simulink library "fixpt_megmaFuncBlkhidden1"  (Simulink 5.0)
libraries: funcsetup x5, fixpt_lib_3p1 x5, fixpt_megmaFuncBlkhidden1 x2
settings Model: Creator=krishnan  LastModifiedBy=krishnan  ExtModeAutoUpdateStatusClock=off

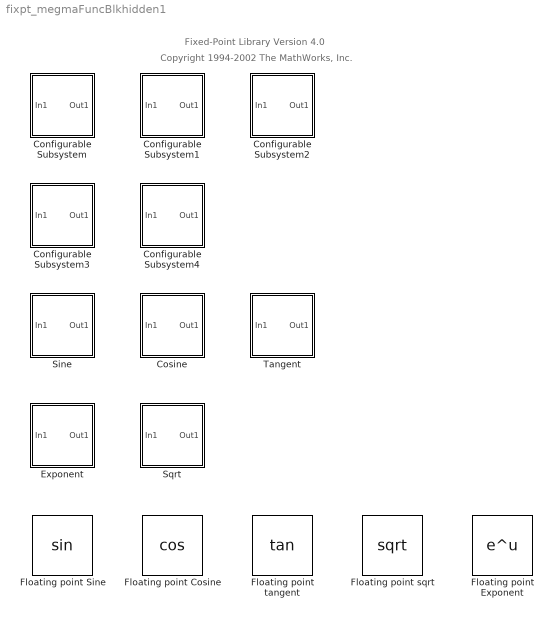
== system fixpt_megmaFuncBlkhidden1 ==
  note: Fixed-Point Library Version 4.0
  note: Copyright 1994-2002 The MathWorks, Inc.
  Configurable Subsystem : Subsystem  BlockChoice=Floating point Sine
      settings: TemplateBlock=self  MemberBlocks=Floating point Sine,Sine
  Configurable Subsystem1 : Subsystem  BlockChoice=Cosine
      settings: TemplateBlock=self  MemberBlocks=Cosine,Floating point Cosine
  Configurable Subsystem2 : Subsystem  BlockChoice=Floating point tangent
      settings: TemplateBlock=self  MemberBlocks=Floating point tangent,Tangent
  Configurable Subsystem3 : Subsystem  BlockChoice=Exponent
      settings: TemplateBlock=self  MemberBlocks=Exponent,Floating point Exponent
  Configurable Subsystem4 : Subsystem  BlockChoice=Floating point sqrt
      settings: TemplateBlock=self  MemberBlocks=Floating point sqrt,Sqrt
  Cosine : Subsystem  mask(MEGMA Fixed-Point Cosine){yData=[1 2 3], xData=[1 2 3], Recompute=Compute always, yData_nonvisible=, xData_nonvisible=, Spacing_nonvisible=, Nptsmax_nonvisible=, ErrMax_nonvisible=, RndMeth_nonvisible=, yScale_nonvisible=, yDt_nonvisible=, xScale_nonvisible=, xDt_nonvisible=, xMax_nonvisible=, xMin_nonvisible=, Spacing='pow2', Nptsmax=[], ErrMax=0.01, RndMeth='floor', yScale=2^-5, xScale=2^-5, yDt=sfix(16), xDt=sfix(16), xmax=2*pi, xmin=0}
      mask prompts: Recompute "Lookup table breakpoints"; Spacing "Allowed spacing 'pow2','even', or 'unrestricted'(default)"; Nptsmax "Maximum number of breakpoints"; ErrMax "Maximum worst case approximation error"; RndMeth "Rounding method 'floor'(default),'ceil','near' or 'zero'"; yScale "Output Scaling"; xScale "Input Scaling"; yDt "Output Datatype"; xDt "Input Datatype"; xmax "Maximum input value of interest"; xmin "Minimum input value of interest"
      mask help: MEGMA Cosine
      mask init:
      | FuncStr = 'cos(x)';
      | if Recompute ~= 3
      |  [xData,yData]= fixpt_look1_func_approx(FuncStr,xmin,xmax,xDt,xScale,yDt,yScale,RndMeth,ErrMax,Nptsmax,Spacing,Recompute);
      | end
      mask Help: web(fpbhelp('cosine'));
      mask StyleString: edit,edit,popup(Compute Always|Cache for a specific MATLAB session|Cache across different MATLAB sessions),edit,edit,edit,edit,edit,edit,edit,edit,edit,edit,edit,edit,edit,edit,edit,edit,edit,edit,edit,edit,edit,edit
      mask Display: disp('y=cos(x)')
  Exponent : Subsystem  mask(MEGMA Fixed-Point Exponent){yData=[1 2 3], xData=[1 2 3], Recompute=Compute always, yData_nonvisible=, xData_nonvisible=, Spacing_nonvisible=, Nptsmax_nonvisible=, ErrMax_nonvisible=, RndMeth_nonvisible=, yScale_nonvisible=, yDt_nonvisible=, xScale_nonvisible=, xDt_nonvisible=, xMax_nonvisible=, xMin_nonvisible=, Spacing='pow2', Nptsmax=[], ErrMax=0.01, RndMeth='floor', yScale=2^-5, xScale=2^-5, yDt=sfix(16), xDt=sfix(16), xmax=2*pi, xmin=0}
      mask prompts: Recompute "Lookup table breakpoints"; Spacing "Allowed spacing 'pow2','even', or 'unrestricted'(default)"; Nptsmax "Maximum number of breakpoints"; ErrMax "Maximum worst case approximation error"; RndMeth "Rounding method 'floor'(default),'ceil','near' or 'zero'"; yScale "Output Scaling"; xScale "Input Scaling"; yDt "Output Datatype"; xDt "Input Datatype"; xmax "Maximum input value of interest"; xmin "Minimum input value of interest"
      mask help: MEGMA Exponent
      mask init:
      | FuncStr = 'exp(x)';
      | if Recompute ~= 3
      |  [xData,yData]= fixpt_look1_func_approx(FuncStr,xmin,xmax,xDt,xScale,yDt,yScale,RndMeth,ErrMax,Nptsmax,Spacing,Recompute);
      | end
      mask Help: web(fpbhelp('exponent'));
      mask StyleString: edit,edit,popup(Compute Always|Cache for a specific MATLAB session|Cache across different MATLAB sessions),edit,edit,edit,edit,edit,edit,edit,edit,edit,edit,edit,edit,edit,edit,edit,edit,edit,edit,edit,edit,edit,edit
      mask Display: disp('y=exp(x)')
  Floating point Cosine : Trigonometry  Operator=cos
  Floating point Exponent : Math
  Floating point Sine : Trigonometry
  Floating point sqrt : Math  Operator=sqrt
  Floating point tangent : Trigonometry  Operator=tan
  Sine : Subsystem  mask(MEGMA Fixed-Point Sine){yData=[1 2 3], xData=[1 2 3], Recompute=Compute always, yData_nonvisible=, xData_nonvisible=, Spacing_nonvisible=, Nptsmax_nonvisible=, ErrMax_nonvisible=, RndMeth_nonvisible=, yScale_nonvisible=, yDt_nonvisible=, xScale_nonvisible=, xDt_nonvisible=, xMax_nonvisible=, xMin_nonvisible=, Spacing='pow2', Nptsmax=[], ErrMax=0.01, RndMeth='floor', yScale=2^-5, xScale=2^-5, yDt=sfix(16), xDt=sfix(16), xmax=2*pi, xmin=0}
      mask prompts: Recompute "Lookup table breakpoints"; Spacing "Allowed spacing 'pow2','even', or 'unrestricted'(default)"; Nptsmax "Maximum number of breakpoints"; ErrMax "Maximum worst case approximation error"; RndMeth "Rounding method 'floor'(default),'ceil','near' or 'zero'"; yScale "Output Scaling"; xScale "Input Scaling"; yDt "Output Datatype"; xDt "Input Datatype"; xmax "Maximum input value of interest"; xmin "Minimum input value of interest"
      mask help: MEGMA Sine
      mask init:
      | FuncStr = 'sin(x)';
      | if Recompute ~= 3
      |  [xData,yData]= fixpt_look1_func_approx(FuncStr,xmin,xmax,xDt,xScale,yDt,yScale,RndMeth,ErrMax,Nptsmax,Spacing,Recompute);
      | end
      mask Help: web(fpbhelp('sine'));
      mask StyleString: edit,edit,popup(Compute Always|Cache for a specific MATLAB session|Cache across different MATLAB sessions),edit,edit,edit,edit,edit,edit,edit,edit,edit,edit,edit,edit,edit,edit,edit,edit,edit,edit,edit,edit,edit,edit
      mask Display: disp('y=sin(x)')
  Sqrt : Subsystem  mask(MEGMA Fixed-Point Sqrt){yData=[1 2 3], xData=[1 2 3], Recompute=Compute always, yData_nonvisible=, xData_nonvisible=, Spacing_nonvisible=, Nptsmax_nonvisible=, ErrMax_nonvisible=, RndMeth_nonvisible=, yScale_nonvisible=, yDt_nonvisible=, xScale_nonvisible=, xDt_nonvisible=, xMax_nonvisible=, xMin_nonvisible=, Spacing='pow2', Nptsmax=[], ErrMax=0.01, RndMeth='floor', yScale=2^-5, xScale=2^-5, yDt=sfix(16), xDt=sfix(16), xmax=2*pi, xmin=0}
      mask prompts: Recompute "Lookup table breakpoints"; Spacing "Allowed spacing 'pow2','even', or 'unrestricted'(default)"; Nptsmax "Maximum number of breakpoints"; ErrMax "Maximum worst case approximation error"; RndMeth "Rounding method 'floor'(default),'ceil','near' or 'zero'"; yScale "Output Scaling"; xScale "Input Scaling"; yDt "Output Datatype"; xDt "Input Datatype"; xmax "Maximum input value of interest"; xmin "Minimum input value of interest"
      mask help: MEGMA Sqrt
      mask init:
      | FuncStr = 'sqrt(x)';
      | if Recompute ~= 3
      |  [xData,yData]= fixpt_look1_func_approx(FuncStr,xmin,xmax,xDt,xScale,yDt,yScale,RndMeth,ErrMax,Nptsmax,Spacing,Recompute);
      | end
      mask Help: web(fpbhelp('sqrt'));
      mask StyleString: edit,edit,popup(Compute Always|Cache for a specific MATLAB session|Cache across different MATLAB sessions),edit,edit,edit,edit,edit,edit,edit,edit,edit,edit,edit,edit,edit,edit,edit,edit,edit,edit,edit,edit,edit,edit
      mask Display: disp('y=sqrt(x)')
  Tangent : Subsystem  mask(MEGMA Fixed-Point Tangent){yData=[1 2 3], xData=[1 2 3], Recompute=Compute always, yData_nonvisible=, xData_nonvisible=, Spacing_nonvisible=, Nptsmax_nonvisible=, ErrMax_nonvisible=, RndMeth_nonvisible=, yScale_nonvisible=, yDt_nonvisible=, xScale_nonvisible=, xDt_nonvisible=, xMax_nonvisible=, xMin_nonvisible=, Spacing='pow2', Nptsmax=[], ErrMax=0.01, RndMeth='floor', yScale=2^-5, xScale=2^-5, yDt=sfix(16), xDt=sfix(16), xmax=2*pi, xmin=0}
      mask prompts: Recompute "Lookup table breakpoints"; Spacing "Allowed spacing 'pow2','even', or 'unrestricted'(default)"; Nptsmax "Maximum number of breakpoints"; ErrMax "Maximum worst case approximation error"; RndMeth "Rounding method 'floor'(default),'ceil','near' or 'zero'"; yScale "Output Scaling"; xScale "Input Scaling"; yDt "Output Datatype"; xDt "Input Datatype"; xmax "Maximum input value of interest"; xmin "Minimum input value of interest"
      mask help: MEGMA Tangent
      mask init:
      | FuncStr = 'tan(x)';
      | if Recompute ~= 3
      |  [xData,yData]= fixpt_look1_func_approx(FuncStr,xmin,xmax,xDt,xScale,yDt,yScale,RndMeth,ErrMax,Nptsmax,Spacing,Recompute);
      | end
      mask Help: web(fpbhelp('tangent'));
      mask StyleString: edit,edit,popup(Compute Always|Cache for a specific MATLAB session|Cache across different MATLAB sessions),edit,edit,edit,edit,edit,edit,edit,edit,edit,edit,edit,edit,edit,edit,edit,edit,edit,edit,edit,edit,edit,edit
      mask Display: disp('y=tan(x)')

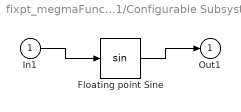
== system fixpt_megmaFuncBlkhidden1/Configurable Subsystem ==
  In1 : Inport
  Floating point Sine : Trigonometry
  Out1 : Outport
  wires:
  In1/1 -> Floating point Sine/1
  Floating point Sine/1 -> Out1/1

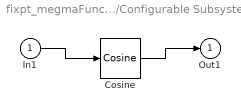
== system fixpt_megmaFuncBlkhidden1/Configurable Subsystem1 ==
  In1 : Inport
  Cosine : fixpt_megmaFuncBlkhidden1/Cosine  yData=[1 2 3]  xData=[1 2 3]  Recompute=Compute Always  yData_nonvisible=[1;0.999511758485136;0.998047510700099;0.995608686458002;0.992197667229329;0.987817783816472;0.982473313101255;0.976169473868635;0.968912421710645;0.960709243015562;0.951567948048172;0.941497463127881;0.930507621912314;0.918609155794918;0.905813683425936;0.892133699366994;0.877582561890373;0.86217447993488;0.845924499231068;0.828848487609326;0.810963119505218;0.792285859677179;0.772834946152472;0.752629372418066;0.731688868873821;0.71003388356608;0.687685562220505;0.664665727593633;0.640996858163325;0.616702066178912;0.591805075092477;0.566330196393309;0.54030230586814;0.513746819310368;0.486689667701963;0.459157271892304;0.431176516798666;0.402774725153557;0.373979630824533;0.344819351732545;0.315322362395269;0.28551746612222;0.255433766888812;0.225100640916817;0.194547707988987;0.163804802525833;0.132901944452825;0.101869309886441;0.0707372016677029;0.0395360197719658;0.00829623162385838;-0.0229516576536404;-0.0541771350269363;-0.0853497093472792;-0.116438941124852;-0.147414472252418;-0.178246055649492;-0.208903584798109;-0.239357123141322;-0.269576933315742;-0.299533506189574;-0.329197589677777;-0.358540217306233;-0.387532736497014;-0.416146836547142;-0.444354576273508;-0.47212841129696;-0.499441220938929;-0.526266334704305;-0.552577558324725;-0.578349199336833;-0.603556092170533;-0.628173622722739;-0.652177752392634;-0.675545041554953;-0.698252672448376;-0.720278471456692;-0.741600930760952;-0.762199229341495;-0.782053253309314;-0.801143615546934;-0.819451674639598;-0.836959553078294;-0.853650154716842;-0.869507181465984;-0.884515149208199;-0.898659402917676;-0.911926130970699;-0.924302378632464;-0.935776060707157;-0.946335973338945;-0.955971804952348;-0.964674146321316;-0.972434499757186;-0.979245287406521;-0.985099858650763;-0.989992496600445;-0.993918423677641;-0.996873806281181;-0.998855758530109;-0.999862345081687;-0.999892583021229;-0.9989464428219;-0.99702484837355;-0.994129676080546;-0.990263753029502;-0.98543085422867;-0.979635698921714;-0.972883945979446;-0.965182188374036;-0.956537946741083;-0.946959662035847;-0.936456687290796;-0.925039278482532;-0.912718584516998;-0.899506636342767;-0.88541633520302;-0.870461440037704;-0.85465655404816;-0.838017110437342;-0.820559357339561;-0.802300341954454;-0.783257893900684;-0.76345060780562;-0.742897825147999;-0.721619615371299;-0.699636756286272;-0.676970713781757;-0.653643620863612;-0.629678256042204;-0.605098021089583;-0.579926918188046;-0.554189526492417;-0.527910978128915;-0.501116933654064;-0.47383355699759;-0.446087489913793;-0.417905825966321;-0.38931608407177;-0.360346181627922;-0.331024407252887;-0.301379393161745;-0.271440087207671;-0.24123572461485;-0.21079579943078;-0.180150035725827;-0.149328358568183;-0.118360864802541;-0.0872777936610349;-0.0561094972351469;-0.0248864108374021;0.00636097671819611;0.0376021528879766;0.0688066111935807;0.0999438810110212;0.130983557324729;0.161895330417537;0.192649015467599;0.223214582023364;0.253562183327795;0.283662185463226;0.313485196288377;0.343002094139282;0.372184056266098;0.401002586978036;0.429429545468913;0.457437173296176;0.484998121486549;0.512085477241841;0.538672790218836;0.564734098357607;0.590243953233023;0.615177444904708;0.639510226241173;0.663218536694376;0.686279225501496;0.70866977429126;0.730368319072748;0.751353671585211;0.771605339988047;0.791103548870739;0.809829258563201;0.827764183727699;0.844890811214172;0.861192417161521;0.876653083328182;0.891257712636015;0.904992043912346;0.917842665815758;0.929797029932041;0.940843463027505;0.950971178447692;0.960170286650366;0.968431804862477;0.975747665851692;0.982110725803907;0.987514771299061;0.991954525378437;0.995425652697519;0.997924763759387;0.999449418224499;0.999998127293645]  xData_nonvisible=[0;0.03125;0.0625;0.09375;0.125;0.15625;0.1875;0.21875;0.25;0.28125;0.3125;0.34375;0.375;0.40625;0.4375;0.46875;0.5;0.53125;0.5625;0.59375;0.625;0.65625;0.6875;0.71875;0.75;0.78125;0.8125;0.84375;0.875;0.90625;0.9375;0.96875;1;1.03125;1.0625;1.09375;1.125;1.15625;1.1875;1.21875;1.25;1.28125;1.3125;1.34375;1.375;1.40625;1.4375;1.46875;1.5;1.53125;1.5625;1.59375;1.625;1.65625;1.6875;1.71875;1.75;1.78125;1.8125;1.84375;1.875;1.90625;1.9375;1.96875;2;2.03125;2.0625;2.09375;2.125;2.15625;2.1875;2.21875;2.25;2.28125;2.3125;2.34375;2.375;2.40625;2.4375;2.46875;2.5;2.53125;2.5625;2.59375;2.625;2.65625;2.6875;2.71875;2.75;2.78125;2.8125;2.84375;2.875;2.90625;2.9375;2.96875;3;3.03125;3.0625;3.09375;3.125;3.15625;3.1875;3.21875;3.25;3.28125;3.3125;3.34375;3.375;3.40625;3.4375;3.46875;3.5;3.53125;3.5625;3.59375;3.625;3.65625;3.6875;3.71875;3.75;3.78125;3.8125;3.84375;3.875;3.90625;3.9375;3.96875;4;4.03125;4.0625;4.09375;4.125;4.15625;4.1875;4.21875;4.25;4.28125;4.3125;4.34375;4.375;4.40625;4.4375;4.46875;4.5;4.53125;4.5625;4.59375;4.625;4.65625;4.6875;4.71875;4.75;4.78125;4.8125;4.84375;4.875;4.90625;4.9375;4.96875;5;5.03125;5.0625;5.09375;5.125;5.15625;5.1875;5.21875;5.25;5.28125;5.3125;5.34375;5.375;5.40625;5.4375;5.46875;5.5;5.53125;5.5625;5.59375;5.625;5.65625;5.6875;5.71875;5.75;5.78125;5.8125;5.84375;5.875;5.90625;5.9375;5.96875;6;6.03125;6.0625;6.09375;6.125;6.15625;6.1875;6.21875;6.25;6.28125]  Spacing_nonvisible='pow2'  Nptsmax_nonvisible=[]  ErrMax_nonvisible=0.01  RndMeth_nonvisible='floor'  yScale_nonvisible=2^-5  yDt_nonvisible=sfix(16)  xScale_nonvisible=2^-5  xDt_nonvisible=sfix(16)  xMax_nonvisible=2*pi  xMin_nonvisible=0  Spacing='pow2'  Nptsmax=[]  ErrMax=0.01  RndMeth='floor'  yScale=2^-5  xScale=2^-5  yDt=sfix(16)  xDt=sfix(16)  xmax=2*pi  xmin=0
  Out1 : Outport
  wires:
  In1/1 -> Cosine/1
  Cosine/1 -> Out1/1

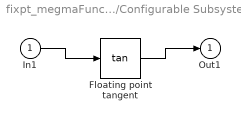
== system fixpt_megmaFuncBlkhidden1/Configurable Subsystem2 ==
  In1 : Inport
  Floating point tangent : Trigonometry  Operator=tan
  Out1 : Outport
  wires:
  In1/1 -> Floating point tangent/1
  Floating point tangent/1 -> Out1/1

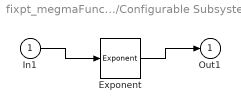
== system fixpt_megmaFuncBlkhidden1/Configurable Subsystem3 ==
  In1 : Inport
  Exponent : fixpt_megmaFuncBlkhidden1/Exponent  yData=[1 2 3]  xData=[1 2 3]  Recompute=Compute Always  yData_nonvisible=[1;1.0317434074991;1.06449445891786;1.09828514030783;1.13314845306683;1.1691184461695;1.20623024942098;1.2445201077661;1.28402541668774;1.32478475872887;1.3668379411738;1.41022603492571;1.4549914146182;1.50117780000012;1.54883029863413;1.59799544995063;1.64872127070013;1.7010573018484;1.7550546569603;1.81076607211939;1.86824595743222;1.92755045016754;1.98873746958229;2.05186677348798;2.11700001661267;2.18420081081562;2.25353478721321;2.32506966027712;2.3988752939671;2.47502376996303;2.55358945806293;2.63464908881563;2.71828182845905;2.80456935623723;2.89359594417176;2.98544853936536;3.08021684891803;3.17799342753884;3.27887376793867;3.38295639409247;3.49034295746184;3.60113833627218;3.7154507379411;3.83339180475841;3.95507672292058;4.08062433502646;4.21015725614396;4.34380199356104;4.48168907033806;4.62395315278208;4.7707331819676;4.92217250943229;5.07841903718008;5.23962536212849;5.40594892514117;5.57755216479126;5.75460267600573;5.93727337374561;6.12574266188199;6.32019460743274;6.52081912033011;6.72781213889469;6.94137582119704;7.16171874249371;7.38905609893065;7.62360991771274;7.86560927394489;8.11529051435645;8.37289748812726;8.6386817850411;8.91290298119874;9.1958288925309;9.48773583635853;9.78890890125589;10.0996422254801;10.4202392842386;10.7510131860764;11.0922869786702;11.4443939643311;11.8076780255212;12.1824939607035;12.5692078308534;12.9681973169691;13.3798520889305;13.8045741860671;14.242778409807;14.6948927287889;15.1613586968345;15.6426318841882;16.1391823224464;16.6514949636101;17.1800701537093;17.7254241214616;18.2880894824436;18.8686157592649;19.4675699182552;20.0855369231877;20.7231203065787;21.3809427591233;22.0596467378412;22.7598950935267;23.4823717181174;24.227782212611;24.9968545761854;25.7903399171931;26.6090131867249;27.4536739354601;28.3251470945409;29.2242837812349;30.1519621301721;31.1090881509677;32.0965966130693;33.1154519586923;34.166649244734;35.2512151145885;36.3702088008095;37.524723159601;38.7158857381472;39.9448598758219;41.2128458403547;42.5210820000628;43.8708460332935;45.2634561762588;46.7002725104795;48.1826982910988;49.7121813173595;51.2902153465857;52.9183415530491;54.5981500331442;56.3312813583435;58.119428177448;59.9643368696996;61.8678092503679;63.8317043304791;65.8579401324037;67.9484955630781;70.1054123466879;72.3307970187014;74.6268229832009;76.9957326355201;79.4398395522613;81.9615307508321;84.563269020706;87.2475953286865;90.0171313005218;92.8745817812945;95.8227374770869;98.8644776805016;102.0027730827;105.240688674702;108.58138674079;112.02812994692;115.584284527188;119.253323571426;123.038830417177;126.944502149322;130.974153210819;135.13171912804;139.421260354375;143.846966235843;148.413159102577;153.124298490199;157.984985495187;162.999967268501;168.174141651845;173.512561961112;179.020441921657;184.703160760245;190.56626845863;196.615491173896;202.856736830865;209.296100892025;215.939872310614;222.794539672674;229.866797534079;237.163552958717;244.69193226422;252.459287981826;260.473206037167;268.741513159002;277.272284523134;286.073851638959;295.154810486372;304.524029910962;314.190660285694;324.164142447555;334.454216917865;345.070933415282;356.024660670779;367.326096554181;378.986278522156;391.016594397853;403.428793492735;416.234998081446;429.447715240934;443.079849065385;457.144713268909;471.656044188264;486.628014198347;502.075245553524;518.012824668342;534.45631685155]  xData_nonvisible=[0;0.03125;0.0625;0.09375;0.125;0.15625;0.1875;0.21875;0.25;0.28125;0.3125;0.34375;0.375;0.40625;0.4375;0.46875;0.5;0.53125;0.5625;0.59375;0.625;0.65625;0.6875;0.71875;0.75;0.78125;0.8125;0.84375;0.875;0.90625;0.9375;0.96875;1;1.03125;1.0625;1.09375;1.125;1.15625;1.1875;1.21875;1.25;1.28125;1.3125;1.34375;1.375;1.40625;1.4375;1.46875;1.5;1.53125;1.5625;1.59375;1.625;1.65625;1.6875;1.71875;1.75;1.78125;1.8125;1.84375;1.875;1.90625;1.9375;1.96875;2;2.03125;2.0625;2.09375;2.125;2.15625;2.1875;2.21875;2.25;2.28125;2.3125;2.34375;2.375;2.40625;2.4375;2.46875;2.5;2.53125;2.5625;2.59375;2.625;2.65625;2.6875;2.71875;2.75;2.78125;2.8125;2.84375;2.875;2.90625;2.9375;2.96875;3;3.03125;3.0625;3.09375;3.125;3.15625;3.1875;3.21875;3.25;3.28125;3.3125;3.34375;3.375;3.40625;3.4375;3.46875;3.5;3.53125;3.5625;3.59375;3.625;3.65625;3.6875;3.71875;3.75;3.78125;3.8125;3.84375;3.875;3.90625;3.9375;3.96875;4;4.03125;4.0625;4.09375;4.125;4.15625;4.1875;4.21875;4.25;4.28125;4.3125;4.34375;4.375;4.40625;4.4375;4.46875;4.5;4.53125;4.5625;4.59375;4.625;4.65625;4.6875;4.71875;4.75;4.78125;4.8125;4.84375;4.875;4.90625;4.9375;4.96875;5;5.03125;5.0625;5.09375;5.125;5.15625;5.1875;5.21875;5.25;5.28125;5.3125;5.34375;5.375;5.40625;5.4375;5.46875;5.5;5.53125;5.5625;5.59375;5.625;5.65625;5.6875;5.71875;5.75;5.78125;5.8125;5.84375;5.875;5.90625;5.9375;5.96875;6;6.03125;6.0625;6.09375;6.125;6.15625;6.1875;6.21875;6.25;6.28125]  Spacing_nonvisible='pow2'  Nptsmax_nonvisible=[]  ErrMax_nonvisible=0.01  RndMeth_nonvisible='floor'  yScale_nonvisible=2^-5  yDt_nonvisible=sfix(16)  xScale_nonvisible=2^-5  xDt_nonvisible=sfix(16)  xMax_nonvisible=2*pi  xMin_nonvisible=0  Spacing='pow2'  Nptsmax=[]  ErrMax=0.01  RndMeth='floor'  yScale=2^-5  xScale=2^-5  yDt=sfix(16)  xDt=sfix(16)  xmax=2*pi  xmin=0
  Out1 : Outport
  wires:
  In1/1 -> Exponent/1
  Exponent/1 -> Out1/1

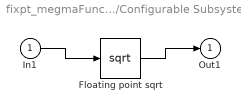
== system fixpt_megmaFuncBlkhidden1/Configurable Subsystem4 ==
  In1 : Inport
  Floating point sqrt : Math  Operator=sqrt
  Out1 : Outport
  wires:
  In1/1 -> Floating point sqrt/1
  Floating point sqrt/1 -> Out1/1

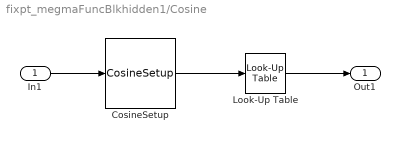
== system fixpt_megmaFuncBlkhidden1/Cosine ==
  In1 : Inport
  CosineSetup : funcsetup/CosineSetup  yData=yData  xData=xData  yData_nonvisible=yData_nonvisible  xData_nonvisible=xData_nonvisible  Spacing_nonvisible=Spacing_nonvisible  Nptsmax_nonvisible=Nptsmax_nonvisible  ErrMax_nonvisible=ErrMax_nonvisible  RndMeth_nonvisible=RndMeth_nonvisible  yScale_nonvisible=yScale_nonvisible  yDt_nonvisible=yDt_nonvisible  xScale_nonvisible=xScale_nonvisible  xDt_nonvisible=xDt_nonvisible  xMax_nonvisible=xMax_nonvisible  xMin_nonvisible=xMin_nonvisible  Spacing=Spacing  Nptsmax=Nptsmax  ErrMax=ErrMax  RndMeth=RndMeth  yScale=yScale  xScale=xScale  yDt=yDt  xDt=xDt  xmax=xmax  xmin=xmin
  Look-Up Table : fixpt_lib_3p1/LookUp/Look-Up Table  XLookUpData=xData  YLookUpData=yData  LookUpMeth=Interpolation-Use End Values  OutputDataTypeScalingMode=Specify via dialog  OutDataType=yDt  OutScaling=yScale  DoSatur=off  DblOver=off  dolog=on
  Out1 : Outport
  wires:
  CosineSetup/1 -> Look-Up Table/1
  In1/1 -> CosineSetup/1
  Look-Up Table/1 -> Out1/1

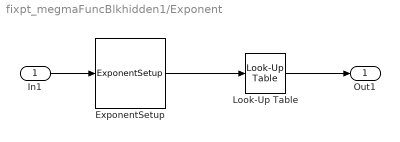
== system fixpt_megmaFuncBlkhidden1/Exponent ==
  In1 : Inport
  ExponentSetup : funcsetup/ExponentSetup  yData=yData  xData=xData  yData_nonvisible=yData_nonvisible  xData_nonvisible=xData_nonvisible  Spacing_nonvisible=Spacing_nonvisible  Nptsmax_nonvisible=Nptsmax_nonvisible  ErrMax_nonvisible=ErrMax_nonvisible  RndMeth_nonvisible=RndMeth_nonvisible  yScale_nonvisible=yScale_nonvisible  yDt_nonvisible=yDt_nonvisible  xScale_nonvisible=xScale_nonvisible  xDt_nonvisible=xDt_nonvisible  xMax_nonvisible=xMax_nonvisible  xMin_nonvisible=xMin_nonvisible  Spacing=Spacing  Nptsmax=Nptsmax  ErrMax=ErrMax  RndMeth=RndMeth  yScale=yScale  xScale=xScale  yDt=yDt  xDt=xDt  xmax=xmax  xmin=xmin
  Look-Up Table : fixpt_lib_3p1/LookUp/Look-Up Table  XLookUpData=xData  YLookUpData=yData  LookUpMeth=Interpolation-Use End Values  OutputDataTypeScalingMode=Specify via dialog  OutDataType=yDt  OutScaling=yScale  DoSatur=off  DblOver=off  dolog=on
  Out1 : Outport
  wires:
  ExponentSetup/1 -> Look-Up Table/1
  In1/1 -> ExponentSetup/1
  Look-Up Table/1 -> Out1/1

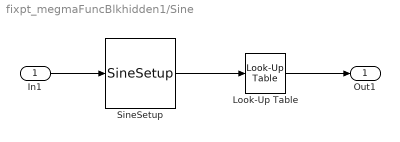
== system fixpt_megmaFuncBlkhidden1/Sine ==
  In1 : Inport
  Look-Up Table : fixpt_lib_3p1/LookUp/Look-Up Table  XLookUpData=xData  YLookUpData=yData  LookUpMeth=Interpolation-Use End Values  OutputDataTypeScalingMode=Specify via dialog  OutDataType=yDt  OutScaling=yScale  DoSatur=off  DblOver=off  dolog=on
  SineSetup : funcsetup/SineSetup  yData=yData  xData=xData  yData_nonvisible=yData_nonvisible  xData_nonvisible=xData_nonvisible  Spacing_nonvisible=Spacing_nonvisible  Nptsmax_nonvisible=Nptsmax_nonvisible  ErrMax_nonvisible=ErrMax_nonvisible  RndMeth_nonvisible=RndMeth_nonvisible  yScale_nonvisible=yScale_nonvisible  yDt_nonvisible=yDt_nonvisible  xScale_nonvisible=xScale_nonvisible  xDt_nonvisible=xDt_nonvisible  xMax_nonvisible=xMax_nonvisible  xMin_nonvisible=xMin_nonvisible  Spacing=Spacing  Nptsmax=Nptsmax  ErrMax=ErrMax  RndMeth=RndMeth  yScale=yScale  xScale=xScale  yDt=yDt  xDt=xDt  xmax=xmax  xmin=xmin
  Out1 : Outport
  wires:
  Look-Up Table/1 -> Out1/1
  In1/1 -> SineSetup/1
  SineSetup/1 -> Look-Up Table/1

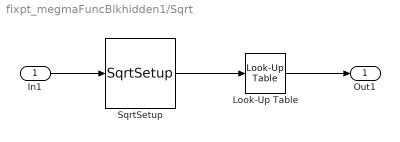
== system fixpt_megmaFuncBlkhidden1/Sqrt ==
  In1 : Inport
  Look-Up Table : fixpt_lib_3p1/LookUp/Look-Up Table  XLookUpData=xData  YLookUpData=yData  LookUpMeth=Interpolation-Use End Values  OutputDataTypeScalingMode=Specify via dialog  OutDataType=yDt  OutScaling=yScale  DoSatur=off  DblOver=off  dolog=on
  SqrtSetup : funcsetup/SqrtSetup  yData=yData  xData=xData  yData_nonvisible=yData_nonvisible  xData_nonvisible=xData_nonvisible  Spacing_nonvisible=Spacing_nonvisible  Nptsmax_nonvisible=Nptsmax_nonvisible  ErrMax_nonvisible=ErrMax_nonvisible  RndMeth_nonvisible=RndMeth_nonvisible  yScale_nonvisible=yScale_nonvisible  yDt_nonvisible=yDt_nonvisible  xScale_nonvisible=xScale_nonvisible  xDt_nonvisible=xDt_nonvisible  xMax_nonvisible=xMax_nonvisible  xMin_nonvisible=xMin_nonvisible  Spacing=Spacing  Nptsmax=Nptsmax  ErrMax=ErrMax  RndMeth=RndMeth  yScale=yScale  xScale=xScale  yDt=yDt  xDt=xDt  xmax=xmax  xmin=xmin
  Out1 : Outport
  wires:
  Look-Up Table/1 -> Out1/1
  In1/1 -> SqrtSetup/1
  SqrtSetup/1 -> Look-Up Table/1

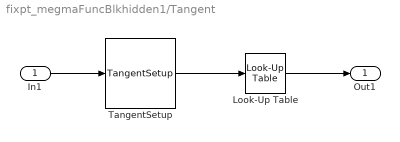
== system fixpt_megmaFuncBlkhidden1/Tangent ==
  In1 : Inport
  Look-Up Table : fixpt_lib_3p1/LookUp/Look-Up Table  XLookUpData=xData  YLookUpData=yData  LookUpMeth=Interpolation-Use End Values  OutputDataTypeScalingMode=Specify via dialog  OutDataType=yDt  OutScaling=yScale  DoSatur=off  DblOver=off  dolog=on
  TangentSetup : funcsetup/TangentSetup  yData=yData  xData=xData  yData_nonvisible=yData_nonvisible  xData_nonvisible=xData_nonvisible  Spacing_nonvisible=Spacing_nonvisible  Nptsmax_nonvisible=Nptsmax_nonvisible  ErrMax_nonvisible=ErrMax_nonvisible  RndMeth_nonvisible=RndMeth_nonvisible  yScale_nonvisible=yScale_nonvisible  yDt_nonvisible=yDt_nonvisible  xScale_nonvisible=xScale_nonvisible  xDt_nonvisible=xDt_nonvisible  xMax_nonvisible=xMax_nonvisible  xMin_nonvisible=xMin_nonvisible  Spacing=Spacing  Nptsmax=Nptsmax  ErrMax=ErrMax  RndMeth=RndMeth  yScale=yScale  xScale=xScale  yDt=yDt  xDt=xDt  xmax=xmax  xmin=xmin
  Out1 : Outport
  wires:
  Look-Up Table/1 -> Out1/1
  In1/1 -> TangentSetup/1
  TangentSetup/1 -> Look-Up Table/1
